simulink model "GPESTN1"  (Simulink 6.1)
settings: Solver=ode45  StartTime=0.0  StopTime=1000.0  MaxStep=0.02  MinStep=0.005  RelTol=1e-3
values from neighbouring files (symbols this model uses):
  A_gpe = 2    [data_GPE.m]    (also in data_GPI.m)
  A_stn = 5    [data_GPI.m]    (also in data_STN.m)
  B_gpe = .08    (= 0.08)    [data_GPE.m]    (also in data_GPI.m)
  B_stn = 1    [data_GPI.m]    (also in data_STN.m)
  c_gpe = 1    [data_GPE.m]
  c_stn = 1    [data_STN.m]
  cag0 = i_v_16(177:192)    [launch_sysGPESTN1.m]    (also in launch_sysGPESTN1_GPEDBS.m)
  cas0 = i_v_16(65:80)    [launch_sysGPESTN1.m]    (also in launch_sysGPESTN1_GPEDBS.m)
  egpegpe = -80    [data_synapses.m]
  egpestn = -100    [data_synapses.m]
  ek_gpe = -80.0    (= -80)    [data_GPE.m]
  ek_stn = -80.0    (= -80)    [data_STN.m]
  el_gpe = -55.0    (= -55)    [data_GPE.m]
  el_stn = -60.0    (= -60)    [data_STN.m]
  epsil_gpe = 1*10^-4    (= 0.0001)    [data_GPE.m]
  epsil_stn = 3.75*10^-5    (= 3.75e-05)    [data_STN.m]
  estngpe = 0    [data_synapses.m]
  gahp_gpe = 30.0    (= 30)    [data_GPE.m]
  gahp_stn = 9.0    (= 9)    [data_STN.m]
  gca_gpe = 0.1    [data_GPE.m]
  gca_stn = 0.5    [data_STN.m]
  ggpegpe = .3    (= 0.3)    [data_synapses.m]    (also in launch_sysGPESTN1.m; launch_sysGPESTN1_GPEDBS.m = 0)
  ggpestn = .90    (= 0.9)    [data_synapses.m]
  gk_gpe = 30.0    (= 30)    [data_GPE.m]
  gk_stn = 45.0    (= 45)    [data_STN.m]
  gl_gpe = .1    (= 0.1)    [data_GPE.m]
  gl_stn = 2.25    [data_STN.m]
  gna_gpe = 120    [data_GPE.m]
  gna_stn = 37.5    [data_STN.m]
  gstngpe = .3    (= 0.3)    [data_synapses.m]
  gt_gpe = .5    (= 0.5)    [data_GPE.m]
  gt_stn = 0.5    [data_STN.m]
  hg0 = i_v_16(129:144)    [launch_sysGPESTN1.m]    (also in launch_sysGPESTN1_GPEDBS.m)
  hs0 = i_v_16(17:32)    [launch_sysGPESTN1.m]    (also in launch_sysGPESTN1_GPEDBS.m)
  k1_gpe = 30.0    (= 30)    [data_GPE.m]
  k1_stn = 15.0    (= 15)    [data_STN.m]
  kca_gpe = 15    [data_GPE.m]
  kca_stn = 22.5    [data_STN.m]
  ng0 = i_v_16(145:160)    [launch_sysGPESTN1.m]    (also in launch_sysGPESTN1_GPEDBS.m)
  ns0 = i_v_16(33:48)    [launch_sysGPESTN1.m]    (also in launch_sysGPESTN1_GPEDBS.m)
  phih_gpe = 0.05    [data_GPE.m]
  phih_stn = 0.75    [data_STN.m]
  phin_gpe = 0.1    [data_GPE.m]
  phin_stn = 0.75    [data_STN.m]
  phir_gpe = 1    [data_GPE.m]
  phir_stn = 0.5    [data_STN.m]
  rg0 = i_v_16(161:176)    [launch_sysGPESTN1.m]    (also in launch_sysGPESTN1_GPEDBS.m)
  rs0 = i_v_16(49:64)    [launch_sysGPESTN1.m]    (also in launch_sysGPESTN1_GPEDBS.m)
  sg0 = i_v_16(193:208)    [launch_sysGPESTN1.m]    (also in launch_sysGPESTN1_GPEDBS.m)
  sigmaa_gpe = 2    [data_GPE.m]
  sigmaa_stn = 7.8    [data_STN.m]
  sigmab_stn = -0.07    [data_STN.m]
  sigmagh_gpe = 2.0    (= 2)    [data_GPE.m]
  sigmagh_stn = 8.0    (= 8)    [data_STN.m]
  sigmah_gpe = -12    [data_GPE.m]
  sigmah_stn = -3.1    [data_STN.m]
  sigmam_gpe = 10.0    (= 10)    [data_GPE.m]
  sigmam_stn = 15.0    (= 15)    [data_STN.m]
  sigman_gpe = 14.0    (= 14)    [data_GPE.m]
  sigman_stn = 8.0    (= 8)    [data_STN.m]
  sigmar_gpe = -2.0    (= -2)    [data_GPE.m]
  sigmar_stn = -2.0    (= -2)    [data_STN.m]
  sigmas_gpe = 2    [data_GPE.m]
  sigmas_stn = 8.0    (= 8)    [data_STN.m]
  sigmatauh_gpe = -12    [data_GPE.m]
  sigmatauh_stn = -3.0    (= -3)    [data_STN.m]
  sigmataun_gpe = -12.0    (= -12)    [data_GPE.m]
  sigmataun_stn = -26.0    (= -26)    [data_STN.m]
  sigmataur_stn = -2.2    [data_STN.m]
  ss0 = i_v_16(81:96)    [launch_sysGPESTN1.m]    (also in launch_sysGPESTN1_GPEDBS.m)
  syn_stngpe_gain = .2    (= 0.2)    [data_STN.m]
  tauh0_gpe = .05    (= 0.05)    [data_GPE.m]
  tauh0_stn = 1.0    (= 1)    [data_STN.m]
  tauh1_gpe = .27    (= 0.27)    [data_GPE.m]
  tauh1_stn = 500.0    (= 500)    [data_STN.m]
  taun0_gpe = .05    (= 0.05)    [data_GPE.m]
  taun0_stn = 1.0    (= 1)    [data_STN.m]
  taun1_gpe = .27    (= 0.27)    [data_GPE.m]
  taun1_stn = 100.0    (= 100)    [data_STN.m]
  taur0_stn = 7.1    [data_STN.m]
  taur1_stn = 17.5    [data_STN.m]
  taur_gpe = 30.0    (= 30)    [data_GPE.m]
  theta_gpe = 20    [data_GPE.m]    (also in data_GPI.m)
  theta_stn = 30    [data_GPI.m]    (also in data_STN.m)
  thetaa_gpe = -57.0    (= -57)    [data_GPE.m]
  thetaa_stn = -63.0    (= -63)    [data_STN.m]
  thetab_stn = 0.25    [data_STN.m]
  thetagh_gpe = -57.0    (= -57)    [data_GPE.m]
  thetagh_stn = -39.0    (= -39)    [data_STN.m]
  thetah_gpe = -58.0    (= -58)    [data_GPE.m]
  thetah_stn = -39.0    (= -39)    [data_STN.m]
  thetam_gpe = -37.0    (= -37)    [data_GPE.m]
  thetam_stn = -30.0    (= -30)    [data_STN.m]
  thetan_gpe = -50.0    (= -50)    [data_GPE.m]
  thetan_stn = -32.0    (= -32)    [data_STN.m]
  thetar_gpe = -70.0    (= -70)    [data_GPE.m]
  thetar_stn = -67.0    (= -67)    [data_STN.m]
  thetas_gpe = -35.0    (= -35)    [data_GPE.m]
  thetas_stn = -39.0    (= -39)    [data_STN.m]
  thetatauh_gpe = -40.0    (= -40)    [data_GPE.m]
  thetatauh_stn = -57.0    (= -57)    [data_STN.m]
  thetataun_gpe = -40.0    (= -40)    [data_GPE.m]
  thetataun_stn = -80.0    (= -80)    [data_STN.m]
  thetataur_stn = 68.0    (= 68)    [data_STN.m]
  vg0 = i_v_16(113:128)    [launch_sysGPESTN1.m]    (also in launch_sysGPESTN1_GPEDBS.m)
  vs0 = i_v_16(1:16)    [launch_sysGPESTN1.m]    (also in launch_sysGPESTN1_GPEDBS.m)
undefined symbols (not defined in the file or in its folder): cag01, cas01, hg01, hs01, ng01, ns01, rg01, rs01, sg01, ss01, vg01, vs01
(part 4 of 9)

== system GPESTN1/STN_cell6/synap_stn ==
  In1 : Inport  Port=1  LatchInput=off
  In4 : Inport  Port=2  LatchInput=off
  Fcn : Fcn  Expr=1/(1+exp(-(u-theta_stn-thetagh_stn)/sigmagh_stn))
  Fcn2 : Fcn  Orientation=left  Expr=A_stn*(1-u)
  Gain : Gain  Orientation=left  Gain=B_stn  SaturateOnIntegerOverflow=on
  Integrator : Integrator  InitialConditionSource=external  InitialCondition=ss01
  Product : Product  SaturateOnIntegerOverflow=on  InputSameDT=on
  Sum : Sum  Inputs=|+-  SaturateOnIntegerOverflow=on  InputSameDT=on
  Out1 : Outport
  wires:
  Fcn/1 -> Product/1
  Fcn2/1 -> Product/2
  Product/1 -> Sum/1
  Sum/1 -> Integrator/1
  Integrator/1 -> Gain/1, Fcn2/1, Out1/1
  Gain/1 -> Sum/2
  In1/1 -> Fcn/1
  In4/1 -> Integrator/2

== system GPESTN1/STN_cell7/Subsystem ==
  In1 : Inport  Port=1  LatchInput=off
  In2 : Inport  Port=2  LatchInput=off
  In3 : Inport  Port=3  LatchInput=off
  In4 : Inport  Port=4  LatchInput=off
  Constant : Constant  Value=vs0
  Constant1 : Constant  Value=ns0
  Constant2 : Constant  Value=hs0
  Constant3 : Constant  Value=rs0
  Constant4 : Constant  Value=cas0
  Gain : Gain  Gain=1/c_stn  SaturateOnIntegerOverflow=on
  Integrator : Integrator  InitialConditionSource=external  InitialCondition=vs01  LimitOutput=on  UpperSaturationLimit=80
  Selector{,1..4} (5 alike) : Selector  IndexMode=Zero-based  ElementSrc=External  Elements=[1 3]
  Sum : Sum  Description=--------  Inputs=-------++  SaturateOnIntegerOverflow=on  InputSameDT=on
  iahp : Subsystem
  ica : Subsystem
  ik : Subsystem
  il : Fcn  Orientation=left  Expr=gl_stn*(u-el_stn)
  ina : Subsystem
  it : Subsystem
  Out1 : Outport
  wires:
  Gain/1 -> Integrator/1
  Sum/1 -> Gain/1
  Integrator/1 -> il/1, ik/1(In1), ina/1(In2), it/1(In2), ica/1(In1), iahp/3(In3), Out1/1
  il/1 -> Sum/1
  ik/1(Out1) -> Sum/2
  ina/1(Out1) -> Sum/3
  ica/1(Out1) -> iahp/2(In2), Sum/5
  it/1(Out1) -> iahp/1(In1), Sum/4
  iahp/1(Out1) -> Sum/6
  In1/1 -> Sum/7
  In2/1 -> Sum/8
  In3/1 -> Sum/9
  Constant4/1 -> Selector4/1
  Constant3/1 -> Selector3/1
  Constant2/1 -> Selector2/1
  Constant1/1 -> Selector1/1
  Constant/1 -> Selector/1
  Selector/1 -> Integrator/2
  Selector1/1 -> ik/2(In2)
  Selector2/1 -> ina/2(In1)
  Selector3/1 -> it/2(In1)
  Selector4/1 -> iahp/4(In4)
  In4/1 -> Selector/2, Selector1/2, Selector2/2, Selector3/2, Selector4/2

== system GPESTN1/STN_cell7/synap_stn ==
  In1 : Inport  Port=1  LatchInput=off
  In4 : Inport  Port=2  LatchInput=off
  Fcn : Fcn  Expr=1/(1+exp(-(u-theta_stn-thetagh_stn)/sigmagh_stn))
  Fcn2 : Fcn  Orientation=left  Expr=A_stn*(1-u)
  Gain : Gain  Orientation=left  Gain=B_stn  SaturateOnIntegerOverflow=on
  Integrator : Integrator  InitialConditionSource=external  InitialCondition=ss01
  Product : Product  SaturateOnIntegerOverflow=on  InputSameDT=on
  Sum : Sum  Inputs=|+-  SaturateOnIntegerOverflow=on  InputSameDT=on
  Out1 : Outport
  wires:
  Fcn/1 -> Product/1
  Fcn2/1 -> Product/2
  Product/1 -> Sum/1
  Sum/1 -> Integrator/1
  Integrator/1 -> Gain/1, Fcn2/1, Out1/1
  Gain/1 -> Sum/2
  In1/1 -> Fcn/1
  In4/1 -> Integrator/2

== system GPESTN1/STN_cell8/Subsystem ==
  In1 : Inport  Port=1  LatchInput=off
  In2 : Inport  Port=2  LatchInput=off
  In3 : Inport  Port=3  LatchInput=off
  In4 : Inport  Port=4  LatchInput=off
  Constant : Constant  Value=vs0
  Constant1 : Constant  Value=ns0
  Constant2 : Constant  Value=hs0
  Constant3 : Constant  Value=rs0
  Constant4 : Constant  Value=cas0
  Gain : Gain  Gain=1/c_stn  SaturateOnIntegerOverflow=on
  Integrator : Integrator  InitialConditionSource=external  InitialCondition=vs01  LimitOutput=on  UpperSaturationLimit=80
  Selector{,1..4} (5 alike) : Selector  IndexMode=Zero-based  ElementSrc=External  Elements=[1 3]
  Sum : Sum  Description=--------  Inputs=-------++  SaturateOnIntegerOverflow=on  InputSameDT=on
  iahp : Subsystem
  ica : Subsystem
  ik : Subsystem
  il : Fcn  Orientation=left  Expr=gl_stn*(u-el_stn)
  ina : Subsystem
  it : Subsystem
  Out1 : Outport
  wires:
  Gain/1 -> Integrator/1
  Sum/1 -> Gain/1
  Integrator/1 -> il/1, ik/1(In1), ina/1(In2), it/1(In2), ica/1(In1), iahp/3(In3), Out1/1
  il/1 -> Sum/1
  ik/1(Out1) -> Sum/2
  ina/1(Out1) -> Sum/3
  ica/1(Out1) -> iahp/2(In2), Sum/5
  it/1(Out1) -> iahp/1(In1), Sum/4
  iahp/1(Out1) -> Sum/6
  In1/1 -> Sum/7
  In2/1 -> Sum/8
  In3/1 -> Sum/9
  Constant4/1 -> Selector4/1
  Constant3/1 -> Selector3/1
  Constant2/1 -> Selector2/1
  Constant1/1 -> Selector1/1
  Constant/1 -> Selector/1
  Selector/1 -> Integrator/2
  Selector1/1 -> ik/2(In2)
  Selector2/1 -> ina/2(In1)
  Selector3/1 -> it/2(In1)
  Selector4/1 -> iahp/4(In4)
  In4/1 -> Selector/2, Selector1/2, Selector2/2, Selector3/2, Selector4/2

== system GPESTN1/STN_cell8/synap_stn ==
  In1 : Inport  Port=1  LatchInput=off
  In4 : Inport  Port=2  LatchInput=off
  Fcn : Fcn  Expr=1/(1+exp(-(u-theta_stn-thetagh_stn)/sigmagh_stn))
  Fcn2 : Fcn  Orientation=left  Expr=A_stn*(1-u)
  Gain : Gain  Orientation=left  Gain=B_stn  SaturateOnIntegerOverflow=on
  Integrator : Integrator  InitialConditionSource=external  InitialCondition=ss01
  Product : Product  SaturateOnIntegerOverflow=on  InputSameDT=on
  Sum : Sum  Inputs=|+-  SaturateOnIntegerOverflow=on  InputSameDT=on
  Out1 : Outport
  wires:
  Fcn/1 -> Product/1
  Fcn2/1 -> Product/2
  Product/1 -> Sum/1
  Sum/1 -> Integrator/1
  Integrator/1 -> Gain/1, Fcn2/1, Out1/1
  Gain/1 -> Sum/2
  In1/1 -> Fcn/1
  In4/1 -> Integrator/2

== system GPESTN1/STN_cell9/Subsystem ==
  In1 : Inport  Port=1  LatchInput=off
  In2 : Inport  Port=2  LatchInput=off
  In3 : Inport  Port=3  LatchInput=off
  In4 : Inport  Port=4  LatchInput=off
  Constant : Constant  Value=vs0
  Constant1 : Constant  Value=ns0
  Constant2 : Constant  Value=hs0
  Constant3 : Constant  Value=rs0
  Constant4 : Constant  Value=cas0
  Gain : Gain  Gain=1/c_stn  SaturateOnIntegerOverflow=on
  Integrator : Integrator  InitialConditionSource=external  InitialCondition=vs01  LimitOutput=on  UpperSaturationLimit=80
  Selector{,1..4} (5 alike) : Selector  IndexMode=Zero-based  ElementSrc=External  Elements=[1 3]
  Sum : Sum  Description=--------  Inputs=-------++  SaturateOnIntegerOverflow=on  InputSameDT=on
  iahp : Subsystem
  ica : Subsystem
  ik : Subsystem
  il : Fcn  Orientation=left  Expr=gl_stn*(u-el_stn)
  ina : Subsystem
  it : Subsystem
  Out1 : Outport
  wires:
  Gain/1 -> Integrator/1
  Sum/1 -> Gain/1
  Integrator/1 -> il/1, ik/1(In1), ina/1(In2), it/1(In2), ica/1(In1), iahp/3(In3), Out1/1
  il/1 -> Sum/1
  ik/1(Out1) -> Sum/2
  ina/1(Out1) -> Sum/3
  ica/1(Out1) -> iahp/2(In2), Sum/5
  it/1(Out1) -> iahp/1(In1), Sum/4
  iahp/1(Out1) -> Sum/6
  In1/1 -> Sum/7
  In2/1 -> Sum/8
  In3/1 -> Sum/9
  Constant4/1 -> Selector4/1
  Constant3/1 -> Selector3/1
  Constant2/1 -> Selector2/1
  Constant1/1 -> Selector1/1
  Constant/1 -> Selector/1
  Selector/1 -> Integrator/2
  Selector1/1 -> ik/2(In2)
  Selector2/1 -> ina/2(In1)
  Selector3/1 -> it/2(In1)
  Selector4/1 -> iahp/4(In4)
  In4/1 -> Selector/2, Selector1/2, Selector2/2, Selector3/2, Selector4/2

== system GPESTN1/STN_cell9/synap_stn ==
  In1 : Inport  Port=1  LatchInput=off
  In4 : Inport  Port=2  LatchInput=off
  Fcn : Fcn  Expr=1/(1+exp(-(u-theta_stn-thetagh_stn)/sigmagh_stn))
  Fcn2 : Fcn  Orientation=left  Expr=A_stn*(1-u)
  Gain : Gain  Orientation=left  Gain=B_stn  SaturateOnIntegerOverflow=on
  Integrator : Integrator  InitialConditionSource=external  InitialCondition=ss01
  Product : Product  SaturateOnIntegerOverflow=on  InputSameDT=on
  Sum : Sum  Inputs=|+-  SaturateOnIntegerOverflow=on  InputSameDT=on
  Out1 : Outport
  wires:
  Fcn/1 -> Product/1
  Fcn2/1 -> Product/2
  Product/1 -> Sum/1
  Sum/1 -> Integrator/1
  Integrator/1 -> Gain/1, Fcn2/1, Out1/1
  Gain/1 -> Sum/2
  In1/1 -> Fcn/1
  In4/1 -> Integrator/2

== system GPESTN1/GPE_cell/gpe_cell/iahp ==
  In1 : Inport  Port=1  LatchInput=off
  In2 : Inport  Port=2  LatchInput=off
  In3 : Inport  Port=3  LatchInput=off
  In4 : Inport  Port=4  LatchInput=off
  Fcn : Fcn  Expr=u/(u+k1_gpe)
  Fcn1 : Fcn  Expr=(u-ek_gpe)*gahp_gpe
  Product : Product  SaturateOnIntegerOverflow=on  InputSameDT=on
  Subsystem : Subsystem
  Out1 : Outport
  wires:
  Subsystem/1(Out1) -> Fcn/1
  Fcn1/1 -> Product/2
  Fcn/1 -> Product/1
  In1/1 -> Subsystem/1(In1)
  In2/1 -> Subsystem/2(In2)
  In3/1 -> Fcn1/1
  Product/1 -> Out1/1
  In4/1 -> Subsystem/3(In3)

== system GPESTN1/GPE_cell/gpe_cell/ica ==
  In1 : Inport  Orientation=down  Port=1  LatchInput=off
  ica_gpe : Subsystem
  sinf : Fcn  Expr=1/(1 + exp(-(u-thetas_gpe)/sigmas_gpe))
  Out1 : Outport
  wires:
  sinf/1 -> ica_gpe/2(In2)
  In1/1 -> sinf/1, ica_gpe/1(In1)
  ica_gpe/1(Out1) -> Out1/1

== system GPESTN1/GPE_cell/gpe_cell/ik ==
  In1 : Inport  Port=1  LatchInput=off
  In2 : Inport  Port=2  LatchInput=off
  ik_gpe : Subsystem
  n_gpe : Subsystem
  Out1 : Outport
  wires:
  n_gpe/1(Out1) -> ik_gpe/2(In2)
  In1/1 -> ik_gpe/1(In1), n_gpe/1(In1)
  ik_gpe/1(Out1) -> Out1/1
  In2/1 -> n_gpe/2(In2)

== system GPESTN1/GPE_cell/gpe_cell/ina ==
  In2 : Inport  Port=1  LatchInput=off
  In1 : Inport  Port=2  LatchInput=off
  h_gpe : Subsystem
  ina_gpe : Subsystem
  minf : Fcn  Expr=1/(1 + exp(-(u-thetam_gpe)/sigmam_gpe))
  Out1 : Outport
  wires:
  h_gpe/1(Out1) -> ina_gpe/3(In3)
  minf/1 -> ina_gpe/2(In2)
  In2/1 -> minf/1, h_gpe/1(In1), ina_gpe/1(In1)
  ina_gpe/1(Out1) -> Out1/1
  In1/1 -> h_gpe/2(In2)

== system GPESTN1/GPE_cell/gpe_cell/it ==
  In2 : Inport  Port=1  LatchInput=off
  In1 : Inport  Port=2  LatchInput=off
  Scope16 : Scope
      settings: YMin=-80  YMax=60
  To Workspace : ToWorkspace  VariableName=rgpe  SampleTime=-1  SaveFormat=Structure
  ainf : Fcn  Expr=1/(1 + exp(-(u-thetaa_gpe)/sigmaa_gpe))
  it_gpe : Subsystem
  r_gpe : Subsystem
  Out1 : Outport
  wires:
  ainf/1 -> it_gpe/3(In3)
  In2/1 -> r_gpe/1(In1), ainf/1, it_gpe/1(In1)
  it_gpe/1(Out1) -> Out1/1
  r_gpe/1(Out1) -> it_gpe/2(In2), To Workspace/1, Scope16/1
  In1/1 -> r_gpe/2(In2)

== system GPESTN1/GPE_cell1/gpe_cell/iahp ==
  In1 : Inport  Port=1  LatchInput=off
  In2 : Inport  Port=2  LatchInput=off
  In3 : Inport  Port=3  LatchInput=off
  In4 : Inport  Port=4  LatchInput=off
  Fcn : Fcn  Expr=u/(u+k1_gpe)
  Fcn1 : Fcn  Expr=(u-ek_gpe)*gahp_gpe
  Product : Product  SaturateOnIntegerOverflow=on  InputSameDT=on
  Subsystem : Subsystem
  Out1 : Outport
  wires:
  Subsystem/1(Out1) -> Fcn/1
  Fcn1/1 -> Product/2
  Fcn/1 -> Product/1
  In1/1 -> Subsystem/1(In1)
  In2/1 -> Subsystem/2(In2)
  In3/1 -> Fcn1/1
  Product/1 -> Out1/1
  In4/1 -> Subsystem/3(In3)

== system GPESTN1/GPE_cell1/gpe_cell/ica ==
  In1 : Inport  Orientation=down  Port=1  LatchInput=off
  ica_gpe : Subsystem
  sinf : Fcn  Expr=1/(1 + exp(-(u-thetas_gpe)/sigmas_gpe))
  Out1 : Outport
  wires:
  sinf/1 -> ica_gpe/2(In2)
  In1/1 -> sinf/1, ica_gpe/1(In1)
  ica_gpe/1(Out1) -> Out1/1

== system GPESTN1/GPE_cell1/gpe_cell/ik ==
  In1 : Inport  Port=1  LatchInput=off
  In2 : Inport  Port=2  LatchInput=off
  ik_gpe : Subsystem
  n_gpe : Subsystem
  Out1 : Outport
  wires:
  n_gpe/1(Out1) -> ik_gpe/2(In2)
  In1/1 -> ik_gpe/1(In1), n_gpe/1(In1)
  ik_gpe/1(Out1) -> Out1/1
  In2/1 -> n_gpe/2(In2)

== system GPESTN1/GPE_cell1/gpe_cell/ina ==
  In2 : Inport  Port=1  LatchInput=off
  In1 : Inport  Port=2  LatchInput=off
  h_gpe : Subsystem
  ina_gpe : Subsystem
  minf : Fcn  Expr=1/(1 + exp(-(u-thetam_gpe)/sigmam_gpe))
  Out1 : Outport
  wires:
  h_gpe/1(Out1) -> ina_gpe/3(In3)
  minf/1 -> ina_gpe/2(In2)
  In2/1 -> minf/1, h_gpe/1(In1), ina_gpe/1(In1)
  ina_gpe/1(Out1) -> Out1/1
  In1/1 -> h_gpe/2(In2)

== system GPESTN1/GPE_cell1/gpe_cell/it ==
  In2 : Inport  Port=1  LatchInput=off
  In1 : Inport  Port=2  LatchInput=off
  ainf : Fcn  Expr=1/(1 + exp(-(u-thetaa_gpe)/sigmaa_gpe))
  it_gpe : Subsystem
  r_gpe : Subsystem
  Out1 : Outport
  wires:
  ainf/1 -> it_gpe/3(In3)
  In2/1 -> r_gpe/1(In1), ainf/1, it_gpe/1(In1)
  it_gpe/1(Out1) -> Out1/1
  r_gpe/1(Out1) -> it_gpe/2(In2)
  In1/1 -> r_gpe/2(In2)

== system GPESTN1/GPE_cell10/gpe_cell/iahp ==
  In1 : Inport  Port=1  LatchInput=off
  In2 : Inport  Port=2  LatchInput=off
  In3 : Inport  Port=3  LatchInput=off
  In4 : Inport  Port=4  LatchInput=off
  Fcn : Fcn  Expr=u/(u+k1_gpe)
  Fcn1 : Fcn  Expr=(u-ek_gpe)*gahp_gpe
  Product : Product  SaturateOnIntegerOverflow=on  InputSameDT=on
  Subsystem : Subsystem
  Out1 : Outport
  wires:
  Subsystem/1(Out1) -> Fcn/1
  Fcn1/1 -> Product/2
  Fcn/1 -> Product/1
  In1/1 -> Subsystem/1(In1)
  In2/1 -> Subsystem/2(In2)
  In3/1 -> Fcn1/1
  Product/1 -> Out1/1
  In4/1 -> Subsystem/3(In3)

== system GPESTN1/GPE_cell10/gpe_cell/ica ==
  In1 : Inport  Orientation=down  Port=1  LatchInput=off
  ica_gpe : Subsystem
  sinf : Fcn  Expr=1/(1 + exp(-(u-thetas_gpe)/sigmas_gpe))
  Out1 : Outport
  wires:
  sinf/1 -> ica_gpe/2(In2)
  In1/1 -> sinf/1, ica_gpe/1(In1)
  ica_gpe/1(Out1) -> Out1/1

== system GPESTN1/GPE_cell10/gpe_cell/ik ==
  In1 : Inport  Port=1  LatchInput=off
  In2 : Inport  Port=2  LatchInput=off
  ik_gpe : Subsystem
  n_gpe : Subsystem
  Out1 : Outport
  wires:
  n_gpe/1(Out1) -> ik_gpe/2(In2)
  In1/1 -> ik_gpe/1(In1), n_gpe/1(In1)
  ik_gpe/1(Out1) -> Out1/1
  In2/1 -> n_gpe/2(In2)

== system GPESTN1/GPE_cell10/gpe_cell/ina ==
  In2 : Inport  Port=1  LatchInput=off
  In1 : Inport  Port=2  LatchInput=off
  h_gpe : Subsystem
  ina_gpe : Subsystem
  minf : Fcn  Expr=1/(1 + exp(-(u-thetam_gpe)/sigmam_gpe))
  Out1 : Outport
  wires:
  h_gpe/1(Out1) -> ina_gpe/3(In3)
  minf/1 -> ina_gpe/2(In2)
  In2/1 -> minf/1, h_gpe/1(In1), ina_gpe/1(In1)
  ina_gpe/1(Out1) -> Out1/1
  In1/1 -> h_gpe/2(In2)

== system GPESTN1/GPE_cell10/gpe_cell/it ==
  In2 : Inport  Port=1  LatchInput=off
  In1 : Inport  Port=2  LatchInput=off
  ainf : Fcn  Expr=1/(1 + exp(-(u-thetaa_gpe)/sigmaa_gpe))
  it_gpe : Subsystem
  r_gpe : Subsystem
  Out1 : Outport
  wires:
  ainf/1 -> it_gpe/3(In3)
  In2/1 -> r_gpe/1(In1), ainf/1, it_gpe/1(In1)
  it_gpe/1(Out1) -> Out1/1
  r_gpe/1(Out1) -> it_gpe/2(In2)
  In1/1 -> r_gpe/2(In2)

== system GPESTN1/GPE_cell11/gpe_cell/iahp ==
  In1 : Inport  Port=1  LatchInput=off
  In2 : Inport  Port=2  LatchInput=off
  In3 : Inport  Port=3  LatchInput=off
  In4 : Inport  Port=4  LatchInput=off
  Fcn : Fcn  Expr=u/(u+k1_gpe)
  Fcn1 : Fcn  Expr=(u-ek_gpe)*gahp_gpe
  Product : Product  SaturateOnIntegerOverflow=on  InputSameDT=on
  Subsystem : Subsystem
  Out1 : Outport
  wires:
  Subsystem/1(Out1) -> Fcn/1
  Fcn1/1 -> Product/2
  Fcn/1 -> Product/1
  In1/1 -> Subsystem/1(In1)
  In2/1 -> Subsystem/2(In2)
  In3/1 -> Fcn1/1
  Product/1 -> Out1/1
  In4/1 -> Subsystem/3(In3)

== system GPESTN1/GPE_cell11/gpe_cell/ica ==
  In1 : Inport  Orientation=down  Port=1  LatchInput=off
  ica_gpe : Subsystem
  sinf : Fcn  Expr=1/(1 + exp(-(u-thetas_gpe)/sigmas_gpe))
  Out1 : Outport
  wires:
  sinf/1 -> ica_gpe/2(In2)
  In1/1 -> sinf/1, ica_gpe/1(In1)
  ica_gpe/1(Out1) -> Out1/1

== system GPESTN1/GPE_cell11/gpe_cell/ik ==
  In1 : Inport  Port=1  LatchInput=off
  In2 : Inport  Port=2  LatchInput=off
  ik_gpe : Subsystem
  n_gpe : Subsystem
  Out1 : Outport
  wires:
  n_gpe/1(Out1) -> ik_gpe/2(In2)
  In1/1 -> ik_gpe/1(In1), n_gpe/1(In1)
  ik_gpe/1(Out1) -> Out1/1
  In2/1 -> n_gpe/2(In2)

== system GPESTN1/GPE_cell11/gpe_cell/ina ==
  In2 : Inport  Port=1  LatchInput=off
  In1 : Inport  Port=2  LatchInput=off
  h_gpe : Subsystem
  ina_gpe : Subsystem
  minf : Fcn  Expr=1/(1 + exp(-(u-thetam_gpe)/sigmam_gpe))
  Out1 : Outport
  wires:
  h_gpe/1(Out1) -> ina_gpe/3(In3)
  minf/1 -> ina_gpe/2(In2)
  In2/1 -> minf/1, h_gpe/1(In1), ina_gpe/1(In1)
  ina_gpe/1(Out1) -> Out1/1
  In1/1 -> h_gpe/2(In2)

== system GPESTN1/GPE_cell11/gpe_cell/it ==
  In2 : Inport  Port=1  LatchInput=off
  In1 : Inport  Port=2  LatchInput=off
  ainf : Fcn  Expr=1/(1 + exp(-(u-thetaa_gpe)/sigmaa_gpe))
  it_gpe : Subsystem
  r_gpe : Subsystem
  Out1 : Outport
  wires:
  ainf/1 -> it_gpe/3(In3)
  In2/1 -> r_gpe/1(In1), ainf/1, it_gpe/1(In1)
  it_gpe/1(Out1) -> Out1/1
  r_gpe/1(Out1) -> it_gpe/2(In2)
  In1/1 -> r_gpe/2(In2)

== system GPESTN1/GPE_cell12/gpe_cell/iahp ==
  In1 : Inport  Port=1  LatchInput=off
  In2 : Inport  Port=2  LatchInput=off
  In3 : Inport  Port=3  LatchInput=off
  In4 : Inport  Port=4  LatchInput=off
  Fcn : Fcn  Expr=u/(u+k1_gpe)
  Fcn1 : Fcn  Expr=(u-ek_gpe)*gahp_gpe
  Product : Product  SaturateOnIntegerOverflow=on  InputSameDT=on
  Subsystem : Subsystem
  Out1 : Outport
  wires:
  Subsystem/1(Out1) -> Fcn/1
  Fcn1/1 -> Product/2
  Fcn/1 -> Product/1
  In1/1 -> Subsystem/1(In1)
  In2/1 -> Subsystem/2(In2)
  In3/1 -> Fcn1/1
  Product/1 -> Out1/1
  In4/1 -> Subsystem/3(In3)

== system GPESTN1/GPE_cell12/gpe_cell/ica ==
  In1 : Inport  Orientation=down  Port=1  LatchInput=off
  ica_gpe : Subsystem
  sinf : Fcn  Expr=1/(1 + exp(-(u-thetas_gpe)/sigmas_gpe))
  Out1 : Outport
  wires:
  sinf/1 -> ica_gpe/2(In2)
  In1/1 -> sinf/1, ica_gpe/1(In1)
  ica_gpe/1(Out1) -> Out1/1

== system GPESTN1/GPE_cell12/gpe_cell/ik ==
  In1 : Inport  Port=1  LatchInput=off
  In2 : Inport  Port=2  LatchInput=off
  ik_gpe : Subsystem
  n_gpe : Subsystem
  Out1 : Outport
  wires:
  n_gpe/1(Out1) -> ik_gpe/2(In2)
  In1/1 -> ik_gpe/1(In1), n_gpe/1(In1)
  ik_gpe/1(Out1) -> Out1/1
  In2/1 -> n_gpe/2(In2)

== system GPESTN1/GPE_cell12/gpe_cell/ina ==
  In2 : Inport  Port=1  LatchInput=off
  In1 : Inport  Port=2  LatchInput=off
  h_gpe : Subsystem
  ina_gpe : Subsystem
  minf : Fcn  Expr=1/(1 + exp(-(u-thetam_gpe)/sigmam_gpe))
  Out1 : Outport
  wires:
  h_gpe/1(Out1) -> ina_gpe/3(In3)
  minf/1 -> ina_gpe/2(In2)
  In2/1 -> minf/1, h_gpe/1(In1), ina_gpe/1(In1)
  ina_gpe/1(Out1) -> Out1/1
  In1/1 -> h_gpe/2(In2)

== system GPESTN1/GPE_cell12/gpe_cell/it ==
  In2 : Inport  Port=1  LatchInput=off
  In1 : Inport  Port=2  LatchInput=off
  ainf : Fcn  Expr=1/(1 + exp(-(u-thetaa_gpe)/sigmaa_gpe))
  it_gpe : Subsystem
  r_gpe : Subsystem
  Out1 : Outport
  wires:
  ainf/1 -> it_gpe/3(In3)
  In2/1 -> r_gpe/1(In1), ainf/1, it_gpe/1(In1)
  it_gpe/1(Out1) -> Out1/1
  r_gpe/1(Out1) -> it_gpe/2(In2)
  In1/1 -> r_gpe/2(In2)

== system GPESTN1/GPE_cell13/gpe_cell/iahp ==
  In1 : Inport  Port=1  LatchInput=off
  In2 : Inport  Port=2  LatchInput=off
  In3 : Inport  Port=3  LatchInput=off
  In4 : Inport  Port=4  LatchInput=off
  Fcn : Fcn  Expr=u/(u+k1_gpe)
  Fcn1 : Fcn  Expr=(u-ek_gpe)*gahp_gpe
  Product : Product  SaturateOnIntegerOverflow=on  InputSameDT=on
  Subsystem : Subsystem
  Out1 : Outport
  wires:
  Subsystem/1(Out1) -> Fcn/1
  Fcn1/1 -> Product/2
  Fcn/1 -> Product/1
  In1/1 -> Subsystem/1(In1)
  In2/1 -> Subsystem/2(In2)
  In3/1 -> Fcn1/1
  Product/1 -> Out1/1
  In4/1 -> Subsystem/3(In3)

== system GPESTN1/GPE_cell13/gpe_cell/ica ==
  In1 : Inport  Orientation=down  Port=1  LatchInput=off
  ica_gpe : Subsystem
  sinf : Fcn  Expr=1/(1 + exp(-(u-thetas_gpe)/sigmas_gpe))
  Out1 : Outport
  wires:
  sinf/1 -> ica_gpe/2(In2)
  In1/1 -> sinf/1, ica_gpe/1(In1)
  ica_gpe/1(Out1) -> Out1/1

== system GPESTN1/GPE_cell13/gpe_cell/ik ==
  In1 : Inport  Port=1  LatchInput=off
  In2 : Inport  Port=2  LatchInput=off
  ik_gpe : Subsystem
  n_gpe : Subsystem
  Out1 : Outport
  wires:
  n_gpe/1(Out1) -> ik_gpe/2(In2)
  In1/1 -> ik_gpe/1(In1), n_gpe/1(In1)
  ik_gpe/1(Out1) -> Out1/1
  In2/1 -> n_gpe/2(In2)

== system GPESTN1/GPE_cell13/gpe_cell/ina ==
  In2 : Inport  Port=1  LatchInput=off
  In1 : Inport  Port=2  LatchInput=off
  h_gpe : Subsystem
  ina_gpe : Subsystem
  minf : Fcn  Expr=1/(1 + exp(-(u-thetam_gpe)/sigmam_gpe))
  Out1 : Outport
  wires:
  h_gpe/1(Out1) -> ina_gpe/3(In3)
  minf/1 -> ina_gpe/2(In2)
  In2/1 -> minf/1, h_gpe/1(In1), ina_gpe/1(In1)
  ina_gpe/1(Out1) -> Out1/1
  In1/1 -> h_gpe/2(In2)

== system GPESTN1/GPE_cell13/gpe_cell/it ==
  In2 : Inport  Port=1  LatchInput=off
  In1 : Inport  Port=2  LatchInput=off
  ainf : Fcn  Expr=1/(1 + exp(-(u-thetaa_gpe)/sigmaa_gpe))
  it_gpe : Subsystem
  r_gpe : Subsystem
  Out1 : Outport
  wires:
  ainf/1 -> it_gpe/3(In3)
  In2/1 -> r_gpe/1(In1), ainf/1, it_gpe/1(In1)
  it_gpe/1(Out1) -> Out1/1
  r_gpe/1(Out1) -> it_gpe/2(In2)
  In1/1 -> r_gpe/2(In2)

== system GPESTN1/GPE_cell14/gpe_cell/iahp ==
  In1 : Inport  Port=1  LatchInput=off
  In2 : Inport  Port=2  LatchInput=off
  In3 : Inport  Port=3  LatchInput=off
  In4 : Inport  Port=4  LatchInput=off
  Fcn : Fcn  Expr=u/(u+k1_gpe)
  Fcn1 : Fcn  Expr=(u-ek_gpe)*gahp_gpe
  Product : Product  SaturateOnIntegerOverflow=on  InputSameDT=on
  Subsystem : Subsystem
  Out1 : Outport
  wires:
  Subsystem/1(Out1) -> Fcn/1
  Fcn1/1 -> Product/2
  Fcn/1 -> Product/1
  In1/1 -> Subsystem/1(In1)
  In2/1 -> Subsystem/2(In2)
  In3/1 -> Fcn1/1
  Product/1 -> Out1/1
  In4/1 -> Subsystem/3(In3)

== system GPESTN1/GPE_cell14/gpe_cell/ica ==
  In1 : Inport  Orientation=down  Port=1  LatchInput=off
  ica_gpe : Subsystem
  sinf : Fcn  Expr=1/(1 + exp(-(u-thetas_gpe)/sigmas_gpe))
  Out1 : Outport
  wires:
  sinf/1 -> ica_gpe/2(In2)
  In1/1 -> sinf/1, ica_gpe/1(In1)
  ica_gpe/1(Out1) -> Out1/1

== system GPESTN1/GPE_cell14/gpe_cell/ik ==
  In1 : Inport  Port=1  LatchInput=off
  In2 : Inport  Port=2  LatchInput=off
  ik_gpe : Subsystem
  n_gpe : Subsystem
  Out1 : Outport
  wires:
  n_gpe/1(Out1) -> ik_gpe/2(In2)
  In1/1 -> ik_gpe/1(In1), n_gpe/1(In1)
  ik_gpe/1(Out1) -> Out1/1
  In2/1 -> n_gpe/2(In2)

== system GPESTN1/GPE_cell14/gpe_cell/ina ==
  In2 : Inport  Port=1  LatchInput=off
  In1 : Inport  Port=2  LatchInput=off
  h_gpe : Subsystem
  ina_gpe : Subsystem
  minf : Fcn  Expr=1/(1 + exp(-(u-thetam_gpe)/sigmam_gpe))
  Out1 : Outport
  wires:
  h_gpe/1(Out1) -> ina_gpe/3(In3)
  minf/1 -> ina_gpe/2(In2)
  In2/1 -> minf/1, h_gpe/1(In1), ina_gpe/1(In1)
  ina_gpe/1(Out1) -> Out1/1
  In1/1 -> h_gpe/2(In2)

== system GPESTN1/GPE_cell14/gpe_cell/it ==
  In2 : Inport  Port=1  LatchInput=off
  In1 : Inport  Port=2  LatchInput=off
  ainf : Fcn  Expr=1/(1 + exp(-(u-thetaa_gpe)/sigmaa_gpe))
  it_gpe : Subsystem
  r_gpe : Subsystem
  Out1 : Outport
  wires:
  ainf/1 -> it_gpe/3(In3)
  In2/1 -> r_gpe/1(In1), ainf/1, it_gpe/1(In1)
  it_gpe/1(Out1) -> Out1/1
  r_gpe/1(Out1) -> it_gpe/2(In2)
  In1/1 -> r_gpe/2(In2)

== system GPESTN1/GPE_cell15/gpe_cell/iahp ==
  In1 : Inport  Port=1  LatchInput=off
  In2 : Inport  Port=2  LatchInput=off
  In3 : Inport  Port=3  LatchInput=off
  In4 : Inport  Port=4  LatchInput=off
  Fcn : Fcn  Expr=u/(u+k1_gpe)
  Fcn1 : Fcn  Expr=(u-ek_gpe)*gahp_gpe
  Product : Product  SaturateOnIntegerOverflow=on  InputSameDT=on
  Subsystem : Subsystem
  Out1 : Outport
  wires:
  Subsystem/1(Out1) -> Fcn/1
  Fcn1/1 -> Product/2
  Fcn/1 -> Product/1
  In1/1 -> Subsystem/1(In1)
  In2/1 -> Subsystem/2(In2)
  In3/1 -> Fcn1/1
  Product/1 -> Out1/1
  In4/1 -> Subsystem/3(In3)

== system GPESTN1/GPE_cell15/gpe_cell/ica ==
  In1 : Inport  Orientation=down  Port=1  LatchInput=off
  ica_gpe : Subsystem
  sinf : Fcn  Expr=1/(1 + exp(-(u-thetas_gpe)/sigmas_gpe))
  Out1 : Outport
  wires:
  sinf/1 -> ica_gpe/2(In2)
  In1/1 -> sinf/1, ica_gpe/1(In1)
  ica_gpe/1(Out1) -> Out1/1

== system GPESTN1/GPE_cell15/gpe_cell/ik ==
  In1 : Inport  Port=1  LatchInput=off
  In2 : Inport  Port=2  LatchInput=off
  ik_gpe : Subsystem
  n_gpe : Subsystem
  Out1 : Outport
  wires:
  n_gpe/1(Out1) -> ik_gpe/2(In2)
  In1/1 -> ik_gpe/1(In1), n_gpe/1(In1)
  ik_gpe/1(Out1) -> Out1/1
  In2/1 -> n_gpe/2(In2)

== system GPESTN1/GPE_cell15/gpe_cell/ina ==
  In2 : Inport  Port=1  LatchInput=off
  In1 : Inport  Port=2  LatchInput=off
  h_gpe : Subsystem
  ina_gpe : Subsystem
  minf : Fcn  Expr=1/(1 + exp(-(u-thetam_gpe)/sigmam_gpe))
  Out1 : Outport
  wires:
  h_gpe/1(Out1) -> ina_gpe/3(In3)
  minf/1 -> ina_gpe/2(In2)
  In2/1 -> minf/1, h_gpe/1(In1), ina_gpe/1(In1)
  ina_gpe/1(Out1) -> Out1/1
  In1/1 -> h_gpe/2(In2)

== system GPESTN1/GPE_cell15/gpe_cell/it ==
  In2 : Inport  Port=1  LatchInput=off
  In1 : Inport  Port=2  LatchInput=off
  ainf : Fcn  Expr=1/(1 + exp(-(u-thetaa_gpe)/sigmaa_gpe))
  it_gpe : Subsystem
  r_gpe : Subsystem
  Out1 : Outport
  wires:
  ainf/1 -> it_gpe/3(In3)
  In2/1 -> r_gpe/1(In1), ainf/1, it_gpe/1(In1)
  it_gpe/1(Out1) -> Out1/1
  r_gpe/1(Out1) -> it_gpe/2(In2)
  In1/1 -> r_gpe/2(In2)

== system GPESTN1/GPE_cell2/gpe_cell/iahp ==
  In1 : Inport  Port=1  LatchInput=off
  In2 : Inport  Port=2  LatchInput=off
  In3 : Inport  Port=3  LatchInput=off
  In4 : Inport  Port=4  LatchInput=off
  Fcn : Fcn  Expr=u/(u+k1_gpe)
  Fcn1 : Fcn  Expr=(u-ek_gpe)*gahp_gpe
  Product : Product  SaturateOnIntegerOverflow=on  InputSameDT=on
  Subsystem : Subsystem
  Out1 : Outport
  wires:
  Subsystem/1(Out1) -> Fcn/1
  Fcn1/1 -> Product/2
  Fcn/1 -> Product/1
  In1/1 -> Subsystem/1(In1)
  In2/1 -> Subsystem/2(In2)
  In3/1 -> Fcn1/1
  Product/1 -> Out1/1
  In4/1 -> Subsystem/3(In3)

== system GPESTN1/GPE_cell2/gpe_cell/ica ==
  In1 : Inport  Orientation=down  Port=1  LatchInput=off
  ica_gpe : Subsystem
  sinf : Fcn  Expr=1/(1 + exp(-(u-thetas_gpe)/sigmas_gpe))
  Out1 : Outport
  wires:
  sinf/1 -> ica_gpe/2(In2)
  In1/1 -> sinf/1, ica_gpe/1(In1)
  ica_gpe/1(Out1) -> Out1/1

== system GPESTN1/GPE_cell2/gpe_cell/ik ==
  In1 : Inport  Port=1  LatchInput=off
  In2 : Inport  Port=2  LatchInput=off
  ik_gpe : Subsystem
  n_gpe : Subsystem
  Out1 : Outport
  wires:
  n_gpe/1(Out1) -> ik_gpe/2(In2)
  In1/1 -> ik_gpe/1(In1), n_gpe/1(In1)
  ik_gpe/1(Out1) -> Out1/1
  In2/1 -> n_gpe/2(In2)

== system GPESTN1/GPE_cell2/gpe_cell/ina ==
  In2 : Inport  Port=1  LatchInput=off
  In1 : Inport  Port=2  LatchInput=off
  h_gpe : Subsystem
  ina_gpe : Subsystem
  minf : Fcn  Expr=1/(1 + exp(-(u-thetam_gpe)/sigmam_gpe))
  Out1 : Outport
  wires:
  h_gpe/1(Out1) -> ina_gpe/3(In3)
  minf/1 -> ina_gpe/2(In2)
  In2/1 -> minf/1, h_gpe/1(In1), ina_gpe/1(In1)
  ina_gpe/1(Out1) -> Out1/1
  In1/1 -> h_gpe/2(In2)

== system GPESTN1/GPE_cell2/gpe_cell/it ==
  In2 : Inport  Port=1  LatchInput=off
  In1 : Inport  Port=2  LatchInput=off
  ainf : Fcn  Expr=1/(1 + exp(-(u-thetaa_gpe)/sigmaa_gpe))
  it_gpe : Subsystem
  r_gpe : Subsystem
  Out1 : Outport
  wires:
  ainf/1 -> it_gpe/3(In3)
  In2/1 -> r_gpe/1(In1), ainf/1, it_gpe/1(In1)
  it_gpe/1(Out1) -> Out1/1
  r_gpe/1(Out1) -> it_gpe/2(In2)
  In1/1 -> r_gpe/2(In2)

== system GPESTN1/GPE_cell3/gpe_cell/iahp ==
  In1 : Inport  Port=1  LatchInput=off
  In2 : Inport  Port=2  LatchInput=off
  In3 : Inport  Port=3  LatchInput=off
  In4 : Inport  Port=4  LatchInput=off
  Fcn : Fcn  Expr=u/(u+k1_gpe)
  Fcn1 : Fcn  Expr=(u-ek_gpe)*gahp_gpe
  Product : Product  SaturateOnIntegerOverflow=on  InputSameDT=on
  Subsystem : Subsystem
  Out1 : Outport
  wires:
  Subsystem/1(Out1) -> Fcn/1
  Fcn1/1 -> Product/2
  Fcn/1 -> Product/1
  In1/1 -> Subsystem/1(In1)
  In2/1 -> Subsystem/2(In2)
  In3/1 -> Fcn1/1
  Product/1 -> Out1/1
  In4/1 -> Subsystem/3(In3)

== system GPESTN1/GPE_cell3/gpe_cell/ica ==
  In1 : Inport  Orientation=down  Port=1  LatchInput=off
  ica_gpe : Subsystem
  sinf : Fcn  Expr=1/(1 + exp(-(u-thetas_gpe)/sigmas_gpe))
  Out1 : Outport
  wires:
  sinf/1 -> ica_gpe/2(In2)
  In1/1 -> sinf/1, ica_gpe/1(In1)
  ica_gpe/1(Out1) -> Out1/1

== system GPESTN1/GPE_cell3/gpe_cell/ik ==
  In1 : Inport  Port=1  LatchInput=off
  In2 : Inport  Port=2  LatchInput=off
  ik_gpe : Subsystem
  n_gpe : Subsystem
  Out1 : Outport
  wires:
  n_gpe/1(Out1) -> ik_gpe/2(In2)
  In1/1 -> ik_gpe/1(In1), n_gpe/1(In1)
  ik_gpe/1(Out1) -> Out1/1
  In2/1 -> n_gpe/2(In2)

== system GPESTN1/GPE_cell3/gpe_cell/ina ==
  In2 : Inport  Port=1  LatchInput=off
  In1 : Inport  Port=2  LatchInput=off
  h_gpe : Subsystem
  ina_gpe : Subsystem
  minf : Fcn  Expr=1/(1 + exp(-(u-thetam_gpe)/sigmam_gpe))
  Out1 : Outport
  wires:
  h_gpe/1(Out1) -> ina_gpe/3(In3)
  minf/1 -> ina_gpe/2(In2)
  In2/1 -> minf/1, h_gpe/1(In1), ina_gpe/1(In1)
  ina_gpe/1(Out1) -> Out1/1
  In1/1 -> h_gpe/2(In2)

== system GPESTN1/GPE_cell3/gpe_cell/it ==
  In2 : Inport  Port=1  LatchInput=off
  In1 : Inport  Port=2  LatchInput=off
  ainf : Fcn  Expr=1/(1 + exp(-(u-thetaa_gpe)/sigmaa_gpe))
  it_gpe : Subsystem
  r_gpe : Subsystem
  Out1 : Outport
  wires:
  ainf/1 -> it_gpe/3(In3)
  In2/1 -> r_gpe/1(In1), ainf/1, it_gpe/1(In1)
  it_gpe/1(Out1) -> Out1/1
  r_gpe/1(Out1) -> it_gpe/2(In2)
  In1/1 -> r_gpe/2(In2)

== system GPESTN1/GPE_cell4/gpe_cell/iahp ==
  In1 : Inport  Port=1  LatchInput=off
  In2 : Inport  Port=2  LatchInput=off
  In3 : Inport  Port=3  LatchInput=off
  In4 : Inport  Port=4  LatchInput=off
  Fcn : Fcn  Expr=u/(u+k1_gpe)
  Fcn1 : Fcn  Expr=(u-ek_gpe)*gahp_gpe
  Product : Product  SaturateOnIntegerOverflow=on  InputSameDT=on
  Subsystem : Subsystem
  Out1 : Outport
  wires:
  Subsystem/1(Out1) -> Fcn/1
  Fcn1/1 -> Product/2
  Fcn/1 -> Product/1
  In1/1 -> Subsystem/1(In1)
  In2/1 -> Subsystem/2(In2)
  In3/1 -> Fcn1/1
  Product/1 -> Out1/1
  In4/1 -> Subsystem/3(In3)

== system GPESTN1/GPE_cell4/gpe_cell/ica ==
  In1 : Inport  Orientation=down  Port=1  LatchInput=off
  ica_gpe : Subsystem
  sinf : Fcn  Expr=1/(1 + exp(-(u-thetas_gpe)/sigmas_gpe))
  Out1 : Outport
  wires:
  sinf/1 -> ica_gpe/2(In2)
  In1/1 -> sinf/1, ica_gpe/1(In1)
  ica_gpe/1(Out1) -> Out1/1

== system GPESTN1/GPE_cell4/gpe_cell/ik ==
  In1 : Inport  Port=1  LatchInput=off
  In2 : Inport  Port=2  LatchInput=off
  ik_gpe : Subsystem
  n_gpe : Subsystem
  Out1 : Outport
  wires:
  n_gpe/1(Out1) -> ik_gpe/2(In2)
  In1/1 -> ik_gpe/1(In1), n_gpe/1(In1)
  ik_gpe/1(Out1) -> Out1/1
  In2/1 -> n_gpe/2(In2)

== system GPESTN1/GPE_cell4/gpe_cell/ina ==
  In2 : Inport  Port=1  LatchInput=off
  In1 : Inport  Port=2  LatchInput=off
  h_gpe : Subsystem
  ina_gpe : Subsystem
  minf : Fcn  Expr=1/(1 + exp(-(u-thetam_gpe)/sigmam_gpe))
  Out1 : Outport
  wires:
  h_gpe/1(Out1) -> ina_gpe/3(In3)
  minf/1 -> ina_gpe/2(In2)
  In2/1 -> minf/1, h_gpe/1(In1), ina_gpe/1(In1)
  ina_gpe/1(Out1) -> Out1/1
  In1/1 -> h_gpe/2(In2)

== system GPESTN1/GPE_cell4/gpe_cell/it ==
  In2 : Inport  Port=1  LatchInput=off
  In1 : Inport  Port=2  LatchInput=off
  ainf : Fcn  Expr=1/(1 + exp(-(u-thetaa_gpe)/sigmaa_gpe))
  it_gpe : Subsystem
  r_gpe : Subsystem
  Out1 : Outport
  wires:
  ainf/1 -> it_gpe/3(In3)
  In2/1 -> r_gpe/1(In1), ainf/1, it_gpe/1(In1)
  it_gpe/1(Out1) -> Out1/1
  r_gpe/1(Out1) -> it_gpe/2(In2)
  In1/1 -> r_gpe/2(In2)

== system GPESTN1/GPE_cell5/gpe_cell/iahp ==
  In1 : Inport  Port=1  LatchInput=off
  In2 : Inport  Port=2  LatchInput=off
  In3 : Inport  Port=3  LatchInput=off
  In4 : Inport  Port=4  LatchInput=off
  Fcn : Fcn  Expr=u/(u+k1_gpe)
  Fcn1 : Fcn  Expr=(u-ek_gpe)*gahp_gpe
  Product : Product  SaturateOnIntegerOverflow=on  InputSameDT=on
  Subsystem : Subsystem
  Out1 : Outport
  wires:
  Subsystem/1(Out1) -> Fcn/1
  Fcn1/1 -> Product/2
  Fcn/1 -> Product/1
  In1/1 -> Subsystem/1(In1)
  In2/1 -> Subsystem/2(In2)
  In3/1 -> Fcn1/1
  Product/1 -> Out1/1
  In4/1 -> Subsystem/3(In3)

== system GPESTN1/GPE_cell5/gpe_cell/ica ==
  In1 : Inport  Orientation=down  Port=1  LatchInput=off
  ica_gpe : Subsystem
  sinf : Fcn  Expr=1/(1 + exp(-(u-thetas_gpe)/sigmas_gpe))
  Out1 : Outport
  wires:
  sinf/1 -> ica_gpe/2(In2)
  In1/1 -> sinf/1, ica_gpe/1(In1)
  ica_gpe/1(Out1) -> Out1/1

== system GPESTN1/GPE_cell5/gpe_cell/ik ==
  In1 : Inport  Port=1  LatchInput=off
  In2 : Inport  Port=2  LatchInput=off
  ik_gpe : Subsystem
  n_gpe : Subsystem
  Out1 : Outport
  wires:
  n_gpe/1(Out1) -> ik_gpe/2(In2)
  In1/1 -> ik_gpe/1(In1), n_gpe/1(In1)
  ik_gpe/1(Out1) -> Out1/1
  In2/1 -> n_gpe/2(In2)

== system GPESTN1/GPE_cell5/gpe_cell/ina ==
  In2 : Inport  Port=1  LatchInput=off
  In1 : Inport  Port=2  LatchInput=off
  h_gpe : Subsystem
  ina_gpe : Subsystem
  minf : Fcn  Expr=1/(1 + exp(-(u-thetam_gpe)/sigmam_gpe))
  Out1 : Outport
  wires:
  h_gpe/1(Out1) -> ina_gpe/3(In3)
  minf/1 -> ina_gpe/2(In2)
  In2/1 -> minf/1, h_gpe/1(In1), ina_gpe/1(In1)
  ina_gpe/1(Out1) -> Out1/1
  In1/1 -> h_gpe/2(In2)

== system GPESTN1/GPE_cell5/gpe_cell/it ==
  In2 : Inport  Port=1  LatchInput=off
  In1 : Inport  Port=2  LatchInput=off
  ainf : Fcn  Expr=1/(1 + exp(-(u-thetaa_gpe)/sigmaa_gpe))
  it_gpe : Subsystem
  r_gpe : Subsystem
  Out1 : Outport
  wires:
  ainf/1 -> it_gpe/3(In3)
  In2/1 -> r_gpe/1(In1), ainf/1, it_gpe/1(In1)
  it_gpe/1(Out1) -> Out1/1
  r_gpe/1(Out1) -> it_gpe/2(In2)
  In1/1 -> r_gpe/2(In2)

== system GPESTN1/GPE_cell6/gpe_cell/iahp ==
  In1 : Inport  Port=1  LatchInput=off
  In2 : Inport  Port=2  LatchInput=off
  In3 : Inport  Port=3  LatchInput=off
  In4 : Inport  Port=4  LatchInput=off
  Fcn : Fcn  Expr=u/(u+k1_gpe)
  Fcn1 : Fcn  Expr=(u-ek_gpe)*gahp_gpe
  Product : Product  SaturateOnIntegerOverflow=on  InputSameDT=on
  Subsystem : Subsystem
  Out1 : Outport
  wires:
  Subsystem/1(Out1) -> Fcn/1
  Fcn1/1 -> Product/2
  Fcn/1 -> Product/1
  In1/1 -> Subsystem/1(In1)
  In2/1 -> Subsystem/2(In2)
  In3/1 -> Fcn1/1
  Product/1 -> Out1/1
  In4/1 -> Subsystem/3(In3)

== system GPESTN1/GPE_cell6/gpe_cell/ica ==
  In1 : Inport  Orientation=down  Port=1  LatchInput=off
  ica_gpe : Subsystem
  sinf : Fcn  Expr=1/(1 + exp(-(u-thetas_gpe)/sigmas_gpe))
  Out1 : Outport
  wires:
  sinf/1 -> ica_gpe/2(In2)
  In1/1 -> sinf/1, ica_gpe/1(In1)
  ica_gpe/1(Out1) -> Out1/1

== system GPESTN1/GPE_cell6/gpe_cell/ik ==
  In1 : Inport  Port=1  LatchInput=off
  In2 : Inport  Port=2  LatchInput=off
  ik_gpe : Subsystem
  n_gpe : Subsystem
  Out1 : Outport
  wires:
  n_gpe/1(Out1) -> ik_gpe/2(In2)
  In1/1 -> ik_gpe/1(In1), n_gpe/1(In1)
  ik_gpe/1(Out1) -> Out1/1
  In2/1 -> n_gpe/2(In2)

== system GPESTN1/GPE_cell6/gpe_cell/ina ==
  In2 : Inport  Port=1  LatchInput=off
  In1 : Inport  Port=2  LatchInput=off
  h_gpe : Subsystem
  ina_gpe : Subsystem
  minf : Fcn  Expr=1/(1 + exp(-(u-thetam_gpe)/sigmam_gpe))
  Out1 : Outport
  wires:
  h_gpe/1(Out1) -> ina_gpe/3(In3)
  minf/1 -> ina_gpe/2(In2)
  In2/1 -> minf/1, h_gpe/1(In1), ina_gpe/1(In1)
  ina_gpe/1(Out1) -> Out1/1
  In1/1 -> h_gpe/2(In2)

== system GPESTN1/GPE_cell6/gpe_cell/it ==
  In2 : Inport  Port=1  LatchInput=off
  In1 : Inport  Port=2  LatchInput=off
  ainf : Fcn  Expr=1/(1 + exp(-(u-thetaa_gpe)/sigmaa_gpe))
  it_gpe : Subsystem
  r_gpe : Subsystem
  Out1 : Outport
  wires:
  ainf/1 -> it_gpe/3(In3)
  In2/1 -> r_gpe/1(In1), ainf/1, it_gpe/1(In1)
  it_gpe/1(Out1) -> Out1/1
  r_gpe/1(Out1) -> it_gpe/2(In2)
  In1/1 -> r_gpe/2(In2)

== system GPESTN1/GPE_cell7/gpe_cell/iahp ==
  In1 : Inport  Port=1  LatchInput=off
  In2 : Inport  Port=2  LatchInput=off
  In3 : Inport  Port=3  LatchInput=off
  In4 : Inport  Port=4  LatchInput=off
  Fcn : Fcn  Expr=u/(u+k1_gpe)
  Fcn1 : Fcn  Expr=(u-ek_gpe)*gahp_gpe
  Product : Product  SaturateOnIntegerOverflow=on  InputSameDT=on
  Subsystem : Subsystem
  Out1 : Outport
  wires:
  Subsystem/1(Out1) -> Fcn/1
  Fcn1/1 -> Product/2
  Fcn/1 -> Product/1
  In1/1 -> Subsystem/1(In1)
  In2/1 -> Subsystem/2(In2)
  In3/1 -> Fcn1/1
  Product/1 -> Out1/1
  In4/1 -> Subsystem/3(In3)

== system GPESTN1/GPE_cell7/gpe_cell/ica ==
  In1 : Inport  Orientation=down  Port=1  LatchInput=off
  ica_gpe : Subsystem
  sinf : Fcn  Expr=1/(1 + exp(-(u-thetas_gpe)/sigmas_gpe))
  Out1 : Outport
  wires:
  sinf/1 -> ica_gpe/2(In2)
  In1/1 -> sinf/1, ica_gpe/1(In1)
  ica_gpe/1(Out1) -> Out1/1

== system GPESTN1/GPE_cell7/gpe_cell/ik ==
  In1 : Inport  Port=1  LatchInput=off
  In2 : Inport  Port=2  LatchInput=off
  ik_gpe : Subsystem
  n_gpe : Subsystem
  Out1 : Outport
  wires:
  n_gpe/1(Out1) -> ik_gpe/2(In2)
  In1/1 -> ik_gpe/1(In1), n_gpe/1(In1)
  ik_gpe/1(Out1) -> Out1/1
  In2/1 -> n_gpe/2(In2)

== system GPESTN1/GPE_cell7/gpe_cell/ina ==
  In2 : Inport  Port=1  LatchInput=off
  In1 : Inport  Port=2  LatchInput=off
  h_gpe : Subsystem
  ina_gpe : Subsystem
  minf : Fcn  Expr=1/(1 + exp(-(u-thetam_gpe)/sigmam_gpe))
  Out1 : Outport
  wires:
  h_gpe/1(Out1) -> ina_gpe/3(In3)
  minf/1 -> ina_gpe/2(In2)
  In2/1 -> minf/1, h_gpe/1(In1), ina_gpe/1(In1)
  ina_gpe/1(Out1) -> Out1/1
  In1/1 -> h_gpe/2(In2)

== system GPESTN1/GPE_cell7/gpe_cell/it ==
  In2 : Inport  Port=1  LatchInput=off
  In1 : Inport  Port=2  LatchInput=off
  ainf : Fcn  Expr=1/(1 + exp(-(u-thetaa_gpe)/sigmaa_gpe))
  it_gpe : Subsystem
  r_gpe : Subsystem
  Out1 : Outport
  wires:
  ainf/1 -> it_gpe/3(In3)
  In2/1 -> r_gpe/1(In1), ainf/1, it_gpe/1(In1)
  it_gpe/1(Out1) -> Out1/1
  r_gpe/1(Out1) -> it_gpe/2(In2)
  In1/1 -> r_gpe/2(In2)

== system GPESTN1/GPE_cell8/gpe_cell/iahp ==
  In1 : Inport  Port=1  LatchInput=off
  In2 : Inport  Port=2  LatchInput=off
  In3 : Inport  Port=3  LatchInput=off
  In4 : Inport  Port=4  LatchInput=off
  Fcn : Fcn  Expr=u/(u+k1_gpe)
  Fcn1 : Fcn  Expr=(u-ek_gpe)*gahp_gpe
  Product : Product  SaturateOnIntegerOverflow=on  InputSameDT=on
  Subsystem : Subsystem
  Out1 : Outport
  wires:
  Subsystem/1(Out1) -> Fcn/1
  Fcn1/1 -> Product/2
  Fcn/1 -> Product/1
  In1/1 -> Subsystem/1(In1)
  In2/1 -> Subsystem/2(In2)
  In3/1 -> Fcn1/1
  Product/1 -> Out1/1
  In4/1 -> Subsystem/3(In3)

== system GPESTN1/GPE_cell8/gpe_cell/ica ==
  In1 : Inport  Orientation=down  Port=1  LatchInput=off
  ica_gpe : Subsystem
  sinf : Fcn  Expr=1/(1 + exp(-(u-thetas_gpe)/sigmas_gpe))
  Out1 : Outport
  wires:
  sinf/1 -> ica_gpe/2(In2)
  In1/1 -> sinf/1, ica_gpe/1(In1)
  ica_gpe/1(Out1) -> Out1/1

== system GPESTN1/GPE_cell8/gpe_cell/ik ==
  In1 : Inport  Port=1  LatchInput=off
  In2 : Inport  Port=2  LatchInput=off
  ik_gpe : Subsystem
  n_gpe : Subsystem
  Out1 : Outport
  wires:
  n_gpe/1(Out1) -> ik_gpe/2(In2)
  In1/1 -> ik_gpe/1(In1), n_gpe/1(In1)
  ik_gpe/1(Out1) -> Out1/1
  In2/1 -> n_gpe/2(In2)

== system GPESTN1/GPE_cell8/gpe_cell/ina ==
  In2 : Inport  Port=1  LatchInput=off
  In1 : Inport  Port=2  LatchInput=off
  h_gpe : Subsystem
  ina_gpe : Subsystem
  minf : Fcn  Expr=1/(1 + exp(-(u-thetam_gpe)/sigmam_gpe))
  Out1 : Outport
  wires:
  h_gpe/1(Out1) -> ina_gpe/3(In3)
  minf/1 -> ina_gpe/2(In2)
  In2/1 -> minf/1, h_gpe/1(In1), ina_gpe/1(In1)
  ina_gpe/1(Out1) -> Out1/1
  In1/1 -> h_gpe/2(In2)

== system GPESTN1/GPE_cell8/gpe_cell/it ==
  In2 : Inport  Port=1  LatchInput=off
  In1 : Inport  Port=2  LatchInput=off
  ainf : Fcn  Expr=1/(1 + exp(-(u-thetaa_gpe)/sigmaa_gpe))
  it_gpe : Subsystem
  r_gpe : Subsystem
  Out1 : Outport
  wires:
  ainf/1 -> it_gpe/3(In3)
  In2/1 -> r_gpe/1(In1), ainf/1, it_gpe/1(In1)
  it_gpe/1(Out1) -> Out1/1
  r_gpe/1(Out1) -> it_gpe/2(In2)
  In1/1 -> r_gpe/2(In2)

== system GPESTN1/GPE_cell9/gpe_cell/iahp ==
  In1 : Inport  Port=1  LatchInput=off
  In2 : Inport  Port=2  LatchInput=off
  In3 : Inport  Port=3  LatchInput=off
  In4 : Inport  Port=4  LatchInput=off
  Fcn : Fcn  Expr=u/(u+k1_gpe)
  Fcn1 : Fcn  Expr=(u-ek_gpe)*gahp_gpe
  Product : Product  SaturateOnIntegerOverflow=on  InputSameDT=on
  Subsystem : Subsystem
  Out1 : Outport
  wires:
  Subsystem/1(Out1) -> Fcn/1
  Fcn1/1 -> Product/2
  Fcn/1 -> Product/1
  In1/1 -> Subsystem/1(In1)
  In2/1 -> Subsystem/2(In2)
  In3/1 -> Fcn1/1
  Product/1 -> Out1/1
  In4/1 -> Subsystem/3(In3)

== system GPESTN1/GPE_cell9/gpe_cell/ica ==
  In1 : Inport  Orientation=down  Port=1  LatchInput=off
  ica_gpe : Subsystem
  sinf : Fcn  Expr=1/(1 + exp(-(u-thetas_gpe)/sigmas_gpe))
  Out1 : Outport
  wires:
  sinf/1 -> ica_gpe/2(In2)
  In1/1 -> sinf/1, ica_gpe/1(In1)
  ica_gpe/1(Out1) -> Out1/1

== system GPESTN1/GPE_cell9/gpe_cell/ik ==
  In1 : Inport  Port=1  LatchInput=off
  In2 : Inport  Port=2  LatchInput=off
  ik_gpe : Subsystem
  n_gpe : Subsystem
  Out1 : Outport
  wires:
  n_gpe/1(Out1) -> ik_gpe/2(In2)
  In1/1 -> ik_gpe/1(In1), n_gpe/1(In1)
  ik_gpe/1(Out1) -> Out1/1
  In2/1 -> n_gpe/2(In2)

== system GPESTN1/GPE_cell9/gpe_cell/ina ==
  In2 : Inport  Port=1  LatchInput=off
  In1 : Inport  Port=2  LatchInput=off
  h_gpe : Subsystem
  ina_gpe : Subsystem
  minf : Fcn  Expr=1/(1 + exp(-(u-thetam_gpe)/sigmam_gpe))
  Out1 : Outport
  wires:
  h_gpe/1(Out1) -> ina_gpe/3(In3)
  minf/1 -> ina_gpe/2(In2)
  In2/1 -> minf/1, h_gpe/1(In1), ina_gpe/1(In1)
  ina_gpe/1(Out1) -> Out1/1
  In1/1 -> h_gpe/2(In2)

== system GPESTN1/GPE_cell9/gpe_cell/it ==
  In2 : Inport  Port=1  LatchInput=off
  In1 : Inport  Port=2  LatchInput=off
  ainf : Fcn  Expr=1/(1 + exp(-(u-thetaa_gpe)/sigmaa_gpe))
  it_gpe : Subsystem
  r_gpe : Subsystem
  Out1 : Outport
  wires:
  ainf/1 -> it_gpe/3(In3)
  In2/1 -> r_gpe/1(In1), ainf/1, it_gpe/1(In1)
  it_gpe/1(Out1) -> Out1/1
  r_gpe/1(Out1) -> it_gpe/2(In2)
  In1/1 -> r_gpe/2(In2)

== system GPESTN1/STN_cell1/Subsystem/iahp ==
  In1 : Inport  Port=1  LatchInput=off
  In2 : Inport  Port=2  LatchInput=off
  In3 : Inport  Port=3  LatchInput=off
  In4 : Inport  Port=4  LatchInput=off
  Fcn : Fcn  Expr=u/(u+k1_stn)
  Fcn1 : Fcn  Expr=(u-ek_stn)*gahp_stn
  Product : Product  SaturateOnIntegerOverflow=on  InputSameDT=on
  Subsystem : Subsystem
  Out1 : Outport
  wires:
  Subsystem/1(Out1) -> Fcn/1
  Fcn1/1 -> Product/2
  Fcn/1 -> Product/1
  In1/1 -> Subsystem/1(In1)
  In2/1 -> Subsystem/2(In2)
  In3/1 -> Fcn1/1
  Product/1 -> Out1/1
  In4/1 -> Subsystem/3(In3)

== system GPESTN1/STN_cell1/Subsystem/ica ==
  In1 : Inport  Orientation=down  Port=1  LatchInput=off
  ica_stn1 : Subsystem
  sinf : Fcn  Expr=1/(1 + exp(-(u-thetas_stn)/sigmas_stn))
  Out1 : Outport
  wires:
  sinf/1 -> ica_stn1/2(In2)
  In1/1 -> sinf/1, ica_stn1/1(In1)
  ica_stn1/1(Out1) -> Out1/1

== system GPESTN1/STN_cell1/Subsystem/ik ==
  In1 : Inport  Port=1  LatchInput=off
  In2 : Inport  Port=2  LatchInput=off
  ik_stn : Subsystem
  n_stn : Subsystem
  Out1 : Outport
  wires:
  n_stn/1(Out1) -> ik_stn/2(In2)
  In1/1 -> ik_stn/1(In1), n_stn/1(In1)
  ik_stn/1(Out1) -> Out1/1
  In2/1 -> n_stn/2(In2)

== system GPESTN1/STN_cell1/Subsystem/ina ==
  In2 : Inport  Port=1  LatchInput=off
  In1 : Inport  Port=2  LatchInput=off
  h_stn : Subsystem
  ina_stn : Subsystem
  minf : Fcn  Expr=1/(1 + exp(-(u-thetam_stn)/sigmam_stn))
  Out1 : Outport
  wires:
  h_stn/1(Out1) -> ina_stn/3(In3)
  minf/1 -> ina_stn/2(In2)
  In2/1 -> minf/1, h_stn/1(In1), ina_stn/1(In1)
  ina_stn/1(Out1) -> Out1/1
  In1/1 -> h_stn/2(In2)

== system GPESTN1/STN_cell1/Subsystem/it ==
  In2 : Inport  Port=1  LatchInput=off
  In1 : Inport  Port=2  LatchInput=off
  ainf : Fcn  Expr=1/(1 + exp(-(u-thetaa_stn)/sigmaa_stn))
  binf : Fcn  Expr=(1/(1 + exp((u-thetab_stn)/sigmab_stn))) - (1/(1 + exp(-thetab_stn/sigmab_stn)))
  it_stn : Subsystem
  r_stn1 : Subsystem
  Out1 : Outport
  wires:
  ainf/1 -> it_stn/3(In3)
  In2/1 -> r_stn1/1(In1), ainf/1, it_stn/1(In1)
  it_stn/1(Out1) -> Out1/1
  r_stn1/1(Out1) -> binf/1
  binf/1 -> it_stn/2(In2)
  In1/1 -> r_stn1/2(In2)

== system GPESTN1/STN_cell10/Subsystem/iahp ==
  In1 : Inport  Port=1  LatchInput=off
  In2 : Inport  Port=2  LatchInput=off
  In3 : Inport  Port=3  LatchInput=off
  In4 : Inport  Port=4  LatchInput=off
  Fcn : Fcn  Expr=u/(u+k1_stn)
  Fcn1 : Fcn  Expr=(u-ek_stn)*gahp_stn
  Product : Product  SaturateOnIntegerOverflow=on  InputSameDT=on
  Subsystem : Subsystem
  Out1 : Outport
  wires:
  Subsystem/1(Out1) -> Fcn/1
  Fcn1/1 -> Product/2
  Fcn/1 -> Product/1
  In1/1 -> Subsystem/1(In1)
  In2/1 -> Subsystem/2(In2)
  In3/1 -> Fcn1/1
  Product/1 -> Out1/1
  In4/1 -> Subsystem/3(In3)

== system GPESTN1/STN_cell10/Subsystem/ica ==
  In1 : Inport  Orientation=down  Port=1  LatchInput=off
  ica_stn1 : Subsystem
  sinf : Fcn  Expr=1/(1 + exp(-(u-thetas_stn)/sigmas_stn))
  Out1 : Outport
  wires:
  sinf/1 -> ica_stn1/2(In2)
  In1/1 -> sinf/1, ica_stn1/1(In1)
  ica_stn1/1(Out1) -> Out1/1

== system GPESTN1/STN_cell10/Subsystem/ik ==
  In1 : Inport  Port=1  LatchInput=off
  In2 : Inport  Port=2  LatchInput=off
  ik_stn : Subsystem
  n_stn : Subsystem
  Out1 : Outport
  wires:
  n_stn/1(Out1) -> ik_stn/2(In2)
  In1/1 -> ik_stn/1(In1), n_stn/1(In1)
  ik_stn/1(Out1) -> Out1/1
  In2/1 -> n_stn/2(In2)

== system GPESTN1/STN_cell10/Subsystem/ina ==
  In2 : Inport  Port=1  LatchInput=off
  In1 : Inport  Port=2  LatchInput=off
  h_stn : Subsystem
  ina_stn : Subsystem
  minf : Fcn  Expr=1/(1 + exp(-(u-thetam_stn)/sigmam_stn))
  Out1 : Outport
  wires:
  h_stn/1(Out1) -> ina_stn/3(In3)
  minf/1 -> ina_stn/2(In2)
  In2/1 -> minf/1, h_stn/1(In1), ina_stn/1(In1)
  ina_stn/1(Out1) -> Out1/1
  In1/1 -> h_stn/2(In2)

== system GPESTN1/STN_cell10/Subsystem/it ==
  In2 : Inport  Port=1  LatchInput=off
  In1 : Inport  Port=2  LatchInput=off
  ainf : Fcn  Expr=1/(1 + exp(-(u-thetaa_stn)/sigmaa_stn))
  binf : Fcn  Expr=(1/(1 + exp((u-thetab_stn)/sigmab_stn))) - (1/(1 + exp(-thetab_stn/sigmab_stn)))
  it_stn : Subsystem
  r_stn1 : Subsystem
  Out1 : Outport
  wires:
  ainf/1 -> it_stn/3(In3)
  In2/1 -> r_stn1/1(In1), ainf/1, it_stn/1(In1)
  it_stn/1(Out1) -> Out1/1
  r_stn1/1(Out1) -> binf/1
  binf/1 -> it_stn/2(In2)
  In1/1 -> r_stn1/2(In2)
